simulink model "Ex4_3J"  (R2016b)
settings: Solver=ode23s  StartTime=0.0  StopTime=5000  RelTol=1e-3
values from neighbouring files (symbols this model uses):
  alpha = 0.005    [ex4_3_init.m]    (also in ex4_5_init.m = 12.87)
  alphaA = 1000/80    (= 12.5)    [ex4_3_init.m]
  J1 = 1.2    [ex4_3_init.m]
  J2 = 10000    [ex4_3_init.m]
  Ke = 220/50/pi    (= 1.40056349921)    [ex4_3_init.m]
  Kp_i = 0.22    [ex4_3_init.m]    (also in ex4_5_init.m = 1000)
  Kp_w = 10000000    [ex4_3_init.m]    (also in ex4_5_init.m = 1000)
  La = 0.002    [ex4_3_init.m]    (also in ex4_5_init.m = 0.235783633842)
  Pnoload = 500    [ex4_3_init.m]
  Ra = 0.05    [ex4_3_init.m]    (also in ex4_5_init.m = 0.1442)
  tau = 20*60    (= 1200)    [ex4_3_init.m]
  tau_u = 0.002    [ex4_3_init.m]
  Ti_i = 5.4    [ex4_3_init.m]    (also in ex4_5_init.m = 50)
  Ti_w = 0.01    [ex4_3_init.m]    (also in ex4_5_init.m = 15)
undefined symbols (not defined in the file or in its folder): sigbuilder_block
settings Model: Creator=Niels  LastModifiedBy=Niels

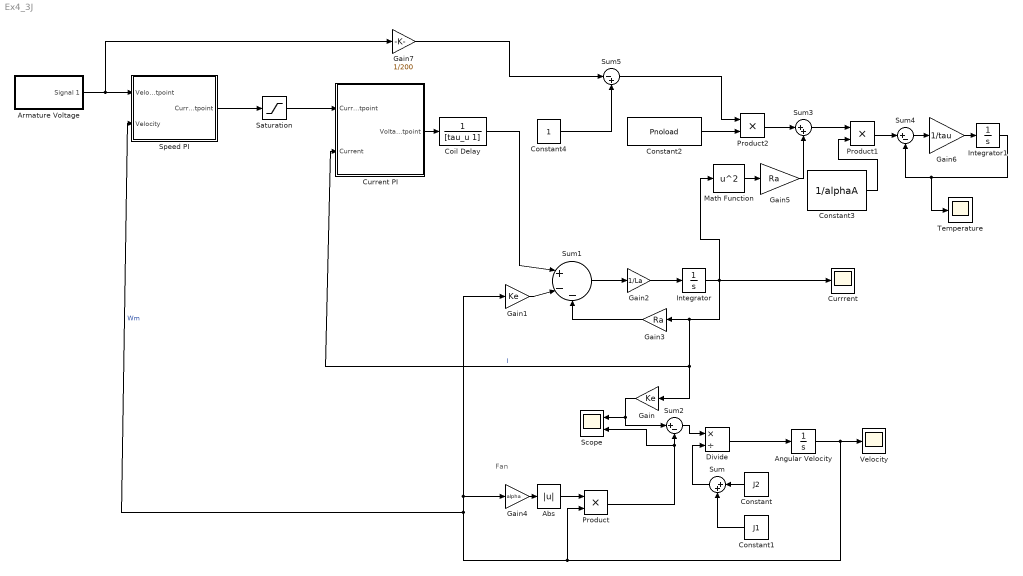
== system Ex4_3J ==
  note: Fan
  Abs : Abs
  Angular Velocity : Integrator
  Armature Voltage : Subsystem  Tag=STV Subsys  LoadFcn=sigbuilder_block('load');  StartFcn=sigbuilder_block('start');  StopFcn=sigbuilder_block('stop');  ClipboardFcn=sigbuilder_block('clipboard');  mask(Sigbuilder block){tuvar=[0:10]}
      mask help: Simulink:masks:SigbuilderBlock_MD
      mask init:
      | if ~strcmp(get_param(bdroot(gcbh),'SimulationStatus'),'stopped') tuvar = sigbuilder_block('maskInit'); end
      settings: CopyFcn=sigbuilder_block('copy');  DeleteFcn=sigbuilder_block('delete');  ModelCloseFcn=sigbuilder_block('modelClose');  PreSaveFcn=sigbuilder_block('preSave');  PauseFcn=sigbuilder_block('pause');  ContinueFcn=sigbuilder_block('continue');  NameChangeFcn=sigbuilder_block('namechange');  OpenFcn=sigbuilder_block('open',[6 30 1428 681.75 ]);  CloseFcn=sigbuilder_block('close');
      mask Display: plot(0, 0, 100, 100,[2, 2, 32, 32, 2], [68, 8, 8, 68, 68],[32, 2], [38, 38], [32, 19, 2],[53, 60, 44], [32, 17, 17, 2],[16, 16, 31, 31]);txt = getActiveGroup(gcbh);text(2, 100, txt,'verticalAlignment', 'top');
  Coil Delay : TransferFcn  Denominator=[tau_u 1]
  Constant : Constant  Value=J2
  Constant1 : Constant  Value=J1
  Constant2 : Constant  Value=Pnoload
  Constant3 : Constant  Value=1/alphaA
  Constant4 : Constant
  Current PI : Subsystem
  Currrent : Scope
  Divide : Product  Inputs=*/
  Gain : Gain  Gain=Ke
  Gain1 : Gain  Gain=Ke
  Gain2 : Gain  Gain=1/La
  Gain3 : Gain  Gain=Ra
  Gain4 : Gain  Gain=alpha
  Gain5 : Gain  Gain=Ra
  Gain6 : Gain  Gain=1/tau
  Gain7 : Gain  Gain=1/200
  Integrator : Integrator
  Integrator1 : Integrator
  Math Function : Math  Operator=square  SaturateOnIntegerOverflow=on
  Product : Product
  Product1 : Product
  Product2 : Product
  Saturation : Saturate  UpperLimit=250  LowerLimit=-250
  Scope : Scope  NumInputPorts=2
  Speed PI : Subsystem
  Sum : Sum  Inputs=|++
  Sum1 : Sum  Inputs=|+--
  Sum2 : Sum  Inputs=|+-
  Sum3 : Sum  Inputs=|++
  Sum4 : Sum  Inputs=|+-
  Sum5 : Sum  Inputs=|-+
  Temperature : Scope
  "Velocity " : Scope
  wires:
  Constant/1 -> Sum/1
  Constant1/1 -> Sum/2
  Sum/1 -> Divide/2
  Gain1/1 -> Sum1/2
  Sum1/1 -> Gain2/1
  Gain2/1 -> Integrator/1
  Integrator/1 -> Math Function/1, Current PI/2(Current), Gain/1, Gain3/1, Currrent/1  "I"
  Gain3/1 -> Sum1/3
  Divide/1 -> Angular Velocity/1
  Sum2/1 -> Divide/1
  Gain4/1 -> Abs/1
  Abs/1 -> Product/1
  Angular Velocity/1 -> "Velocity "/1, Product/2, Speed PI/2(Velocity), Gain1/1, Gain4/1  "Wm"
  Product/1 -> Scope/2, Sum2/2
  Gain/1 -> Scope/1, Sum2/1
  Coil Delay/1 -> Sum1/1
  Armature Voltage/1(Signal 1) -> Gain7/1, Speed PI/1(Velocity Setpoint)
  Current PI/1(Voltage Setpoint) -> Coil Delay/1
  Speed PI/1(Current Setpoint) -> Saturation/1
  Saturation/1 -> Current PI/1(Current Setpoint)
  Constant2/1 -> Product2/2
  Sum3/1 -> Product1/1
  Constant3/1 -> Product1/2
  Gain5/1 -> Sum3/2
  Product1/1 -> Sum4/1
  Sum4/1 -> Gain6/1
  Gain6/1 -> Integrator1/1
  Integrator1/1 -> Temperature/1, Sum4/2
  Math Function/1 -> Gain5/1
  Product2/1 -> Sum3/1
  Sum5/1 -> Product2/1
  Constant4/1 -> Sum5/2
  Gain7/1 -> Sum5/1

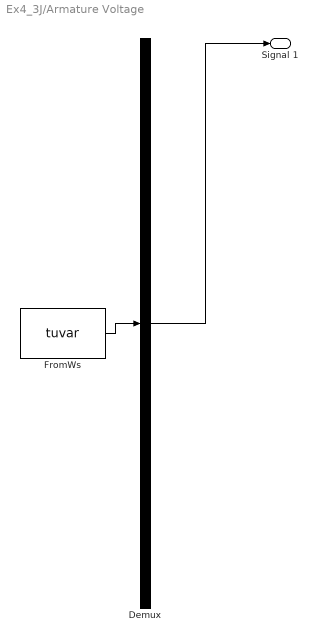
== system Ex4_3J/Armature Voltage ==
  Demux : Demux  Tag=STV Demux  Outputs=1
  FromWs : FromWorkspace  Tag=STV FromWs  VariableName=tuvar  SampleTime=0
      SigBuilderData=|
      | common.afterFinalStr = 'Extrapolate'
      | common.sampleTime = 0
      | dataSet.timeRange = [0 5000]
      | dataSet.name = 'Group 1'
      | sbobj.Groups.Name = 'Group 1'
      | sbobj.Groups.Signals.Name = 'Signal 1'
      | sbobj.Groups.Signals.XData = [0 300 300 900 900 1200 1200 1800 1800 2100 2100 2700 2700 3000 3000 3600 3600 3900 3900 5000]
      | sbobj.Groups.Signals.YData = [200 200 0 0 200 200 0 0 200 200 0 0 200 200 0 0 200 200 0 0]
      | sbobj.Groups.TimeRange = [0 5000]
  Signal 1 : Outport  Tag=STV Outport
  wires:
  Demux/1 -> Signal 1/1
  FromWs/1 -> Demux/1

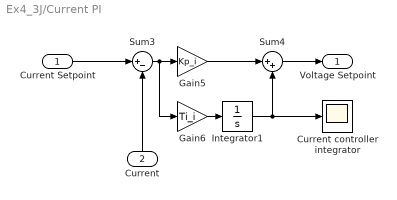
== system Ex4_3J/Current PI ==
  Current Setpoint : Inport
  Current : Inport  Port=2
  Current controller integrator : Scope
  Gain5 : Gain  Gain=Kp_i
  Gain6 : Gain  Gain=Ti_i
  Integrator1 : Integrator
  Sum3 : Sum  Inputs=|+-
  Sum4 : Sum  Inputs=|++
  Voltage Setpoint : Outport
  wires:
  Sum3/1 -> Gain6/1, Gain5/1
  Current Setpoint/1 -> Sum3/1
  Sum4/1 -> Voltage Setpoint/1
  Current/1 -> Sum3/2
  Integrator1/1 -> Current controller integrator/1, Sum4/2
  Gain6/1 -> Integrator1/1
  Gain5/1 -> Sum4/1

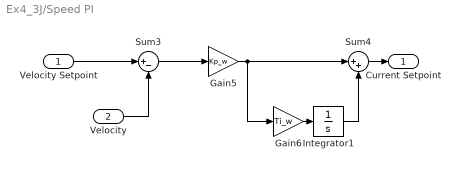
== system Ex4_3J/Speed PI ==
  Velocity Setpoint : Inport
  Velocity : Inport  Port=2
  Gain5 : Gain  Gain=Kp_w
  Gain6 : Gain  Gain=Ti_w
  Integrator1 : Integrator
  Sum3 : Sum  Inputs=|+-
  Sum4 : Sum  Inputs=|++
  Current Setpoint : Outport
  wires:
  Gain6/1 -> Integrator1/1
  Sum4/1 -> Current Setpoint/1
  Velocity/1 -> Sum3/2
  Sum3/1 -> Gain5/1
  Velocity Setpoint/1 -> Sum3/1
  Gain5/1 -> Sum4/1, Gain6/1
  Integrator1/1 -> Sum4/2
